simulink model "Project0"  (R2016b)
settings: Solver=VariableStepAuto  StartTime=0.0  StopTime=200  RelTol=1e-3
libraries: dspvision x2, dspsnks4 x2
settings Model: Creator=zengxiangchen  LastModifiedBy=Queensatoria
settings DebuggingCC: ParameterDowncastMsg=none  ParameterPrecisionLossMsg=none

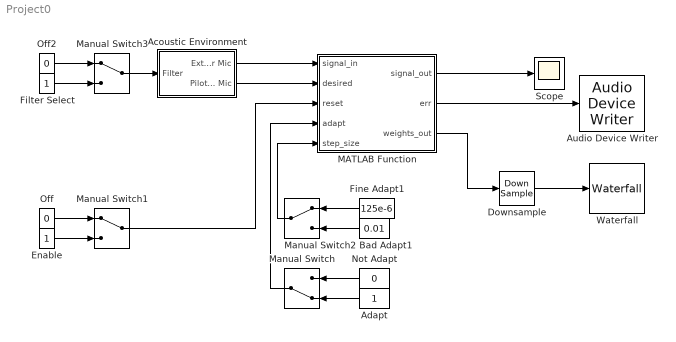
== system Project0 ==
  Acoustic Environment : Subsystem
  Adapt : Constant  OutDataTypeStr=Inherit: Inherit via back propagation
  Audio Device Writer : dspsnks4/Audio Device Writer  Driver=CoreAudio  Device=Default  InheritSampleRate=on  SampleRate=44100  BitDepth=16-bit integer  BufferSize=4096  NumBuffers=10  DefaultOutputChannelMapping=on  OutputChannelMapping=1:2  OutputNumUnderrunSamples=off  DriverIdx=5  DeviceWarnFlag=''
  Bad Adapt1 : Constant  Value=0.01  OutDataTypeStr=Inherit: Inherit via back propagation
  Downsample : DownSample  N=32  RateOptions=Allow multirate processing
  Enable : Constant  OutDataTypeStr=boolean
  Filter Select : Constant  OutDataTypeStr=boolean
  Fine Adapt1 : Constant  Value=125e-6  OutDataTypeStr=Inherit: Inherit via back propagation
  MATLAB Function : MATLAB Function  TreatAsAtomicUnit=on
  Manual Switch : ManualSwitch  CurrentSetting=0
  Manual Switch1 : ManualSwitch
  Manual Switch2 : ManualSwitch
  Manual Switch3 : ManualSwitch
  Not Adapt : Constant  Value=0  OutDataTypeStr=Inherit: Inherit via back propagation
  Off : Constant  Value=0  OutDataTypeStr=boolean
  Off2 : Constant  Value=0  OutDataTypeStr=boolean
  Scope : Scope
  Waterfall : dspsnks4/Waterfall  TraceProperties=off  NumTraces=6  CMapStr=autumn  TNewest=0.9  TOldest=0.5  HistoryLength=50  HistoryFull=Overwrite  UpdateInterval=1  ExportMode=All visible  MLExportName=ExportData  AutoExport=off  DisplayProperties=on  MouseMode=Orbit  AxisGrid=on  Snapshot=off  Suspend=off  SyncSnapshots=off  OpenScopeAtSimStart=off  FigPos=[27 57 405 339]  CameraView=[28.5695107359948 1316.8235109177 -294.350451091202 -0.004386576265097 22.5 3.5 0.594111941595966 -49.3321641526923 11.3523452384532 1.20078102376266 1 86.3856203154502 14.008478970073]  InportDimsHint=[32 1]  AxisProperties=off  AxisColor='w'  XLabel=Samples  YLabel=Amplitude  ZLabel=Time  TriggerProperties=off  TrigStartMode=Immediately  TrigStartT=0  TrigStartN=0  TrigStartFcn=trigbegin  TrigStopMode=Never  TrigStopT=0.1  TrigStopN=1  TrigStopFcn=trigend  TrigRearmMode=Never  TrigRearmT=0  TrigRearmN=0  TrigRearmFcn=trigrearm  XformProperties=off  XformMode=None  XformFcn=abs  XformExpr=(u+1)/2
      settings: YMin=-0.188312025368214  YMax=0.24
  wires:
  Acoustic Environment/1(Exterior Mic) -> MATLAB Function/1(signal_in)
  Acoustic Environment/2(Pilot's Mic) -> MATLAB Function/2(desired)
  Off2/1 -> Manual Switch3/1
  Filter Select/1 -> Manual Switch3/2
  Manual Switch3/1 -> Acoustic Environment/1(Filter)
  MATLAB Function/2(err) -> Audio Device Writer/1
  Downsample/1 -> Waterfall/1
  MATLAB Function/1(signal_out) -> Scope/1
  MATLAB Function/3(weights_out) -> Downsample/1
  Off/1 -> Manual Switch1/1
  Enable/1 -> Manual Switch1/2
  Not Adapt/1 -> Manual Switch/1
  Adapt/1 -> Manual Switch/2
  Manual Switch/1 -> MATLAB Function/4(adapt)
  Manual Switch1/1 -> MATLAB Function/3(reset)
  Fine Adapt1/1 -> Manual Switch2/1
  Bad Adapt1/1 -> Manual Switch2/2
  Manual Switch2/1 -> MATLAB Function/5(step_size)

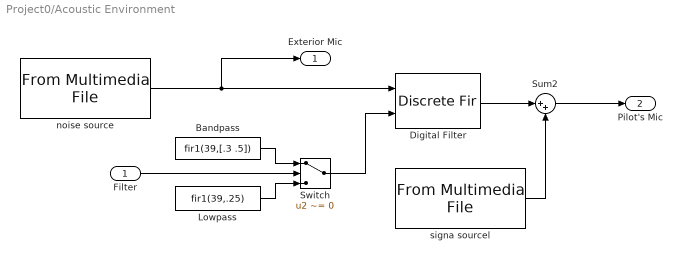
== system Project0/Acoustic Environment ==
  Filter : Inport
  Bandpass : Constant  Value=fir1(39,[.3 .5])  OutDataTypeStr=Inherit: Inherit via back propagation
  Digital Filter : DiscreteFir  CoefSource=Input port  Coefficients=[1 2]  InputProcessing=Columns as channels (frame based)  AccumDataTypeStr=Inherit: Same as product output  OutDataTypeStr=Inherit: Same as input
      settings: InputPortMap=u0,u1
  Lowpass : Constant  Value=fir1(39,.25)  OutDataTypeStr=Inherit: Inherit via back propagation
  Sum2 : Sum  Inputs=|++  SaturateOnIntegerOverflow=on  InputSameDT=on  OutDataTypeStr=Inherit: Same as first input
  Switch : Switch  Criteria=u2 ~= 0  SaturateOnIntegerOverflow=on
  noise source : dspvision/From Multimedia File  inputFilename=/Users/Queensatoria/signal&system/lab5/Noise.wav  loop=on  numPlays=inf  outputStreams=Audio only  videoDataType=single  audioDataType=single  inheritSampleTime=on  userDefinedSampleTime=1/30  noAudioOutput=off  isIntensityVideo=off  fourcc=RGB  colorVideoFormat=Separate color signals  outputEOF=off  dataOrg=Column-major  audioFrameSize=32  computeAudioFrameSize=off  outSamplingMode=Sample based
  signa sourcel : dspvision/From Multimedia File  inputFilename=/Users/Queensatoria/signal&system/lab5/Music.wav  loop=on  numPlays=inf  outputStreams=Audio only  videoDataType=single  audioDataType=single  inheritSampleTime=on  userDefinedSampleTime=1/30  noAudioOutput=off  isIntensityVideo=off  fourcc=RGB  colorVideoFormat=Separate color signals  outputEOF=off  dataOrg=Column-major  audioFrameSize=32  computeAudioFrameSize=off  outSamplingMode=Sample based
  Exterior Mic : Outport
  Pilot's Mic : Outport  Port=2
  wires:
  Sum2/1 -> Pilot's Mic/1
  Filter/1 -> Switch/2
  Digital Filter/1 -> Sum2/1
  Switch/1 -> Digital Filter/2
  Bandpass/1 -> Switch/1
  Lowpass/1 -> Switch/3
  signa sourcel/1 -> Sum2/2
  noise source/1 -> Exterior Mic/1, Digital Filter/1

== matlab function Project0/MATLAB Function ==
  data: signal_in input; desired input; signal_out output; err output; weights_out output; reset input; adapt input; step_size input
function [ signal_out, err, weights_out ] = lms(signal_in, desired, reset, adapt, step_size)
%%%%%%%%%%%%%%%%%%%%%%%%%%%%%%%%%%%%%%%%%%%%%%%%%%%%%%%%%%%%%%%%%%%%%%%%%%%
% Inputs:
%   signal_in:  the pure noise signal captured by Exterior Mic
%   desired:    the input signal mixed with the noise signal(xn)
%   reset:      the switch for resetting the ANC procedure (true for reset)
%   adapt:      the switch for the filter to complete the ANC procedure or not
%   step_size:  a constant which need to adjust to apply the best effect
%
% Outputs:
%   signal_out: the estimated noise
%   err:        music with noise signal - estimated noise
%   weights_out:the weights matrix
%%%%%%%%%%%%%%%%%%%%%%%%%%%%%%%%%%%%%%%%%%%%%%%%%%%%%%%%%%%%%%%%%%%%%%%%%%%

  % Set weights and fifo persisitent to keep the LMS Filter active and affective
  persistent weights;
  persistent fifo;
  % initialization
  signal_out = zeros(length(signal_in),1);  
  err = zeros(length(signal_in),1);
  % get the framesize(32) and the channel number(1) of the input signal,
  % which can be changed if changing the set of microphones
  [ FrameSize,ChannelCount ] = size(signal_in);

      FilterLength = 32;

      mu = step_size;% the parameter we need to adjust by the experiment
        
      if ( reset || isempty(weights) )% the reset usage, the same as the input of LMS Filter of simulink
     
          weights = zeros(FilterLength,1);

          fifo = zeros(FilterLength,ChannelCount);
      end
      
    %the LMS-Filter algorithm is here
    for ch = 1:ChannelCount

       for n = 1:FrameSize
           % iteration to get one new sample and remain the total sample number is 32
           fifo(1:FilterLength-1,ch) = fifo(2:FilterLength,ch);
           fifo(FilterLength,ch) = signal_in(n,ch);
            % yn = wn * xn
            signal_out(n,ch) = weights' * fifo(:,ch);
            % en = dn - yn
            err(n,ch) = desired(n,ch) - signal_out(n,ch) ;
            if adapt % implrment ANC when adapt is true
                % w(n+1) = w(n) + mu * err * fifo
                weights = weights + mu * err(n,ch) * fifo(:,ch);
            end
        end
    end
      weights_out = weights;
end
